simulink model "qcm"  (Simulink 3.00)
undefined symbols (not defined in the file): Double, F64
libraries: mathlib x63, genlib x5, analoglib x5, reglib x1, matrixlib x1, arclib x1
settings Model: MaskType=REX sequence  MaskIconFrame=on  MaskIconOpaque=on  MaskIconRotate=none  MaskIconUnits=autoscale

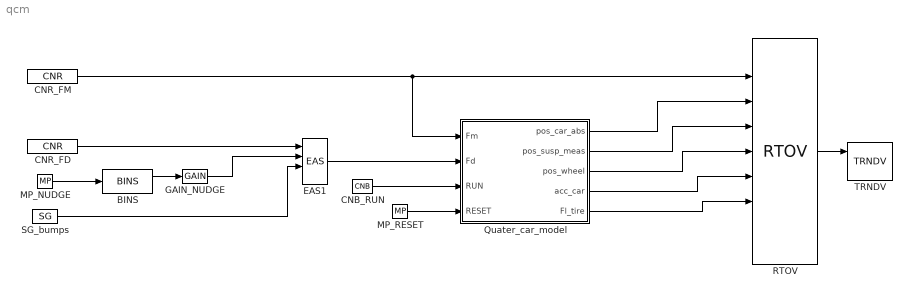
== system qcm ==
  BINS : genlib/BINS  Y0=off  t1=0.1  t2=1  t3=0  t4=4  t5=5  t6=6  t7=7  t8=8  RPT=off
  CNB_RUN : mathlib/CNB  YCN=on
  CNR_FD : mathlib/CNR  ycn=0
  CNR_FM : mathlib/CNR  ycn=0
  EAS1 : mathlib/EAS  a=1  b=1  c=1  d=1  y0=0
  GAIN_NUDGE : mathlib/GAIN  k=1000
  MP_NUDGE : genlib/MP  BSTATE=off  pwidth=0.2  RPTF=off
  MP_RESET : genlib/MP  BSTATE=off  pwidth=1  RPTF=off
  Quater_car_model : Subsystem  mask(REX sequence){k1=44000, noise_amp=1, base_pos_susp=100, base_pos_car=150, k2=500000, b1=1000, b2=200, m1=470, m2=40, m_l=0}
      mask prompts: k1 "stifness c. suspension"; noise_amp "amplitude of susp pos. sensor noise"; base_pos_susp "base measured susp. pos."; base_pos_car "base position of car mass"; k2 "stifness c. tire"; b1 "damping c. suspension"; b2 "damping. c. tire"; m1 "quartercar mass"; m2 "wheel mass"; m_l "additional load mass"
  RTOV : matrixlib/RTOV  nmax=6  offset=0  n=8  etype=8: Double (F64)
  SG_bumps : genlib/SG  isig=4: RANDOM  amp=0  freq=100  phase=0  offset=0  ifrunit=1: Hz  iphunit=1: degrees
  TRNDV : arclib/TRNDV  n=6  l=10000  btype=8: Double (F64)  pfac=1  afac=0  arc=0  id=1  Title=Quater-car model  timesrc=1: CORETIMER  ViewConfig="{\"View\":{\"Data\":{\"History\":20,\"XAxisTimeFormat\":66},\"PropertiesModel\":[{\"Id\":0,\"Items\":[{\"Color\":\"#000099\",\"Id\":0,\"IsActive\":true,\"LineWidth\":2,\"Name\":\"Fm\",\"SceneNumber\":3},{\"Color\":\"#669900\",\"Id\":1,\"IsActive\":true,\"LineWidth\":2,\"Name\":\"pos_car_abs\",\"SceneNumber\":3},{\"Color\":\"#ff0000\",\"Id\":2,\"IsActive\":true,\"LineWidth\":2,\"Name\":\"pos_sus_meas\",\"SceneNumber\":3},{\"Color\":\"#9966cc\",\"Id\":3,\"IsActive\":true,\"LineWidth\":2,\"Name\":\"pos_wheel\",\"SceneNumber\":3},{\"Color\":\"#339999\",\"Id\":4,\"IsActive\":true,\"LineWidth\":2,\"Name\":\"acc_car\",\"SceneNumber\":3},{\"Color\":\"#996600\",\"Id\":5,\"IsActive\":true,\"LineWidth\":2,\"Name\":\"Fl_tire\",\"SceneNumber\":3}]}],\"Scenes\":[{\"Id\":3}],\"sync\":false}}"
  wires:
  BINS/1 -> GAIN_NUDGE/1
  CNB_RUN/1 -> Quater_car_model/3(RUN)
  CNR_FD/1 -> EAS1/1
  CNR_FM/1 -> Quater_car_model/1(Fm), RTOV/2
  EAS1/1 -> Quater_car_model/2(Fd)
  GAIN_NUDGE/1 -> EAS1/2
  MP_NUDGE/1 -> BINS/1
  MP_RESET/1 -> Quater_car_model/4(RESET)
  Quater_car_model/1(pos_car_abs) -> RTOV/3
  Quater_car_model/2(pos_susp_meas) -> RTOV/4
  Quater_car_model/3(pos_wheel) -> RTOV/5
  Quater_car_model/4(acc_car) -> RTOV/6
  Quater_car_model/5(Fl_tire) -> RTOV/7
  RTOV/1 -> TRNDV/1
  SG_bumps/1 -> EAS1/3

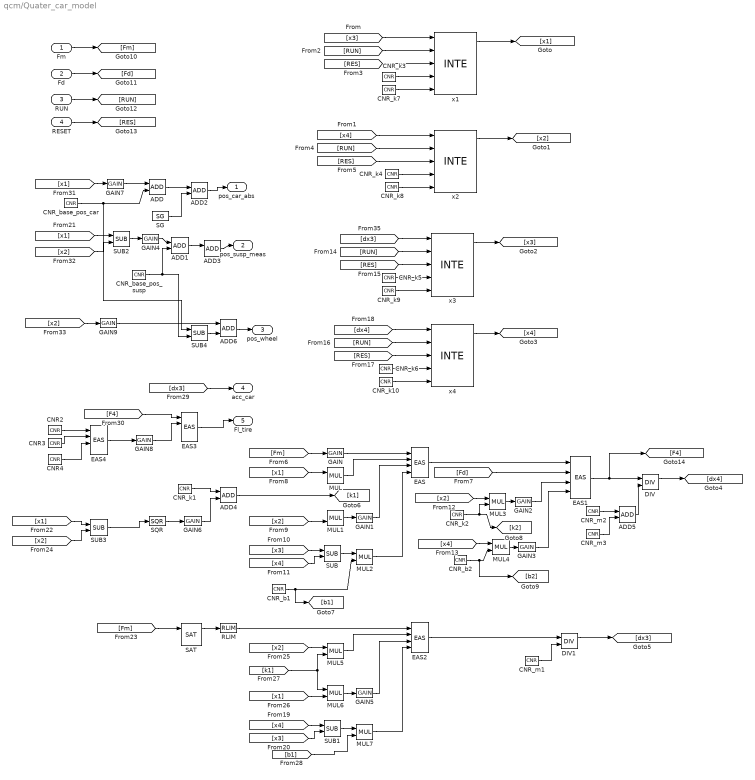
== system qcm/Quater_car_model ==
  Fm : Inport  Port=1
  Fd : Inport  Port=2
  RUN : Inport  Port=3
  RESET : Inport  Port=4
  ADD{,1..6} (7 alike) : mathlib/ADD
  CNR2 : mathlib/CNR  ycn=m1
  CNR3 : mathlib/CNR  ycn=m2
  CNR4 : mathlib/CNR  ycn=m_l
  CNR_b1 : mathlib/CNR  ycn=b1
  CNR_b2 : mathlib/CNR  ycn=b2
  CNR_base_pos_car : mathlib/CNR  ycn=base_pos_car
  CNR_base_pos_susp : mathlib/CNR  ycn=base_pos_susp
  CNR_k1 : mathlib/CNR  ycn=k1
  CNR_k{7..10} (4 alike) : mathlib/CNR  ycn=1
  CNR_k2 : mathlib/CNR  ycn=k2
  CNR_k{3..6} (4 alike) : mathlib/CNR  ycn=0
  CNR_m1 : mathlib/CNR  ycn=m1
  CNR_m2 : mathlib/CNR  ycn=m2
  CNR_m3 : mathlib/CNR  ycn=m_l
  DIV : mathlib/DIV  yerr=1
  DIV1 : mathlib/DIV  yerr=1
  EAS{,1..4} (5 alike) : mathlib/EAS  a=1  b=1  c=1  d=1  y0=0
  GAIN{,1..3,5} (5 alike) : mathlib/GAIN  k=-1
  GAIN4 : mathlib/GAIN  k=1000
  GAIN6 : mathlib/GAIN  k=1e7
  GAIN7 : mathlib/GAIN  k=1000
  GAIN8 : mathlib/GAIN  k=9.81
  GAIN9 : mathlib/GAIN  k=1000
  MUL{,1..7} (8 alike) : mathlib/MUL
  RLIM : analoglib/RLIM  tp=2E-05  tn=2E-05
  SAT : reglib/SAT  tp=1  tn=1  hilim0=5000  lolim0=-5000  HLD=on
  SG : genlib/SG  isig=4: RANDOM  amp=noise_amp  freq=200  phase=0  offset=0  ifrunit=1: Hz  iphunit=1: degrees
  SQR : mathlib/SQR
  SUB{,1..4} (5 alike) : mathlib/SUB
  x1 : analoglib/INTE  ymin=-1  ymax=1  SAT=off
  x2 : analoglib/INTE  ymin=-1  ymax=1  SAT=off
  x3 : analoglib/INTE  ymin=-1e10  ymax=1e10  SAT=off
  x4 : analoglib/INTE  ymin=-1e10  ymax=1e10  SAT=off
  pos_car_abs : Outport  Port=1
  pos_susp_meas : Outport  Port=2
  pos_wheel : Outport  Port=3  OutDataTypeStr=Inherit: auto
  acc_car : Outport  Port=4
  Fl_tire : Outport  Port=5
  wires:
  ADD/1 -> ADD2/1
  ADD1/1 -> ADD3/1
  ADD2/1 -> pos_car_abs/1
  ADD3/1 -> pos_susp_meas/1
  ADD4/1 -> [k1]
  ADD5/1 -> DIV/2
  ADD6/1 -> pos_wheel/1
  CNR2/1 -> EAS4/1
  CNR3/1 -> EAS4/2
  CNR4/1 -> EAS4/3
  CNR_b1/1 -> [b1], MUL2/2
  CNR_b2/1 -> [b2], MUL4/2
  CNR_base_pos_car/1 -> ADD/2, SUB4/1
  CNR_base_pos_susp/1 -> ADD1/2, SUB4/2
  CNR_k1/1 -> ADD4/1
  CNR_k10/1 -> x4/5
  CNR_k2/1 -> [k2], MUL3/2
  CNR_k3/1 -> x1/4
  CNR_k4/1 -> x2/4
  CNR_k5/1 -> x3/4
  CNR_k6/1 -> x4/4
  CNR_k7/1 -> x1/5
  CNR_k8/1 -> x2/5
  CNR_k9/1 -> x3/5
  CNR_m1/1 -> DIV1/2
  CNR_m2/1 -> ADD5/1
  CNR_m3/1 -> ADD5/2
  DIV/1 -> [dx4]
  DIV1/1 -> [dx3]
  EAS/1 -> EAS1/1
  EAS1/1 -> DIV/1, [F4]
  EAS2/1 -> DIV1/1
  EAS3/1 -> Fl_tire/1
  EAS4/1 -> GAIN8/1
  Fd/1 -> [Fd]
  Fm/1 -> [Fm]
  [x3] -> x1/1
  [x4] -> x2/1
  [x3] -> SUB/1
  [x4] -> SUB/2
  [x2] -> MUL3/1
  [x4] -> MUL4/1
  [RUN] -> x3/2
  [RES] -> x3/3
  [RUN] -> x4/2
  [RES] -> x4/3
  [dx4] -> x4/1
  [x4] -> SUB1/1
  [RUN] -> x1/2
  [x3] -> SUB1/2
  [x1] -> SUB2/1
  [x1] -> SUB3/1
  [Fm] -> SAT/1
  [x2] -> SUB3/2
  [x2] -> MUL5/1
  [x1] -> MUL6/2
  [k1] -> MUL5/2, MUL6/1
  [b1] -> MUL7/2
  [dx3] -> acc_car/1
  [RES] -> x1/3
  [F4] -> EAS3/1
  [x1] -> GAIN7/1
  [x2] -> SUB2/2
  [x2] -> GAIN9/1
  [dx3] -> x3/1
  [RUN] -> x2/2
  [RES] -> x2/3
  [Fm] -> GAIN/1
  [Fd] -> EAS1/2
  [x1] -> MUL/1
  [x2] -> MUL1/2
  GAIN/1 -> EAS/1
  GAIN1/1 -> EAS/3
  GAIN2/1 -> EAS1/3
  GAIN3/1 -> EAS1/4
  GAIN4/1 -> ADD1/1
  GAIN5/1 -> EAS2/3
  GAIN6/1 -> ADD4/2
  GAIN7/1 -> ADD/1
  GAIN8/1 -> EAS3/2
  GAIN9/1 -> ADD6/1
  MUL/1 -> EAS/2
  MUL1/1 -> GAIN1/1
  MUL2/1 -> EAS/4
  MUL3/1 -> GAIN2/1
  MUL4/1 -> GAIN3/1
  MUL5/1 -> EAS2/2
  MUL6/1 -> GAIN5/1
  MUL7/1 -> EAS2/4
  RESET/1 -> [RES]
  RLIM/1 -> EAS2/1
  RUN/1 -> [RUN]
  SAT/1 -> RLIM/1
  SG/1 -> ADD2/2
  SQR/1 -> GAIN6/1
  SUB/1 -> MUL2/1
  SUB1/1 -> MUL7/1
  SUB2/1 -> GAIN4/1
  SUB3/1 -> SQR/1
  SUB4/1 -> ADD6/2
  x1/1 -> [x1]
  x2/1 -> [x2]
  x3/1 -> [x3]
  x4/1 -> [x4]
